simulink subsystem "vessel_pressure"  (R2019b)
settings: Solver=VariableStepAuto  StartTime=0.0  StopTime=10.0  RelTol=1e-3
settings Model: Creator=RH  LastModifiedBy=RH

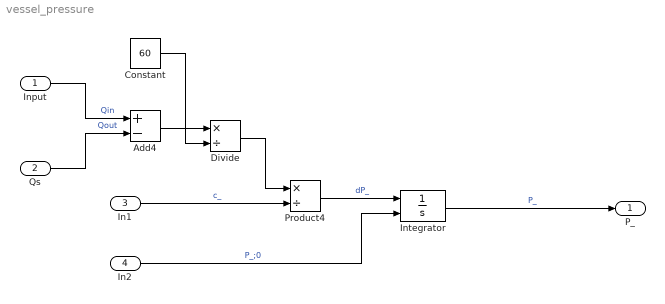
== system vessel_pressure ==
  Input : Inport  Unit=liter/minute
  Qs : Inport  Port=2  Unit=liter/minute
  In1 : Inport  Port=3  Unit=liter/mmHg
  In2 : Inport  Port=4  Unit=mmHg
  Add4 : Sum  Inputs=+-
  Constant : Constant  Value=60
  Divide : Product  Inputs=*/
  Integrator : Integrator  InitialConditionSource=external
  Product4 : Product  Inputs=*/
  P_ : Outport  Unit=mmHg
  wires:
  Divide/1 -> Product4/1
  Qs/1 -> Add4/2  "Qout"
  In1/1 -> Product4/2  "c_"
  In2/1 -> Integrator/2  "P_;0"
  Add4/1 -> Divide/1
  Integrator/1 -> P_/1  "P_"
  Product4/1 -> Integrator/1  "dP_"
  Input/1 -> Add4/1  "Qin"
  Constant/1 -> Divide/2
